simulink model "INTMRStateCtrl"  (R2018b)
settings: Solver=FixedStepDiscrete  StartTime=0.0  StopTime=10.0  FixedStep=0.01  RelTol=1e-3
libraries: StateCtrlLib x1
settings Model: Creator=sn2xws  LastModifiedBy=sn2xws
settings DataIOCC: SaveFormat=StructureWithTime
settings OptimizationCC: DefaultParameterBehavior=Inlined  EnhancedBackFolding=on  PassReuseOutputArgsAs=Individual arguments  ZeroExternalMemoryAtStartup=off  ZeroInternalMemoryAtStartup=off  OptimizeBlockOrder=speed  DifferentSizesBufferReuse=on  OptimizationCustomize=off
settings DebuggingCC: ParameterTunabilityLossMsg=error
settings ModelReferenceCC: ModelReferenceNumInstancesAllowed=Single
settings SFSimCC: MATLABDynamicMemAlloc=off
settings RTWCC: SystemTargetFile=autosar.tlc  GenCodeOnly=on  TemplateMakefile=ert_default_tmf  Description=AUTOSAR  GenerateReport=on  IncludeHyperlinkInReport=on  LaunchReport=on  GenerateTraceInfo=on  GenerateTraceReport=on  GenerateTraceReportSl=on  GenerateTraceReportSf=on  GenerateTraceReportEml=on
settings CodeAppCC: ForceParamTrailComments=on  IgnoreCustomStorageClasses=off  OperatorAnnotations=on  SimulinkDataObjDesc=on  SFDataObjDesc=on  InsertBlockDesc=on
settings STFCustomTargetCC: TargetLangStandard=C99 (ISO)  MultiwordLength=256  ParMdlRefBuildCompliant=on  CompOptLevelCompliant=on  IncludeMdlTerminateFcn=off  CombineOutputUpdateFcns=on  SuppressErrorStatus=on  ERTCustomFileBanners=on  SupportNonFinite=off  SupportComplex=off  SupportContinuousTime=off  SupportNonInlinedSFcns=off  RemoveResetFunc=on  MATLABClassNameForMDSCustomization=Simulink.SoftwareTarget.ERTCustomization  AutosarCompliant=on  UseToolchainInfoCompliant=on  LookupTableObjectStructAxisOrder=2,1,3,4,...  LUTObjectStructOrderEvenSpacing=Size,Table,Breakpoints  SystemTargetFile=autosar.tlc
settings ERTTargetCC: TargetLangStandard=C99 (ISO)  ConcurrentExecutionCompliant=off  IncludeMdlTerminateFcn=off  SuppressErrorStatus=on  SupportNonFinite=off  SupportComplex=off  ModelStepFunctionPrototypeControlCompliant=off  CPPClassGenCompliant=off  AutosarCompliant=on  LookupTableObjectStructAxisOrder=2,1,3,4,...  LUTObjectStructOrderEvenSpacing=Size,Table,Breakpoints  InlinedParameterPlacement=NonHierarchical  ERTCustomFileTemplate=example_file_process.tlc

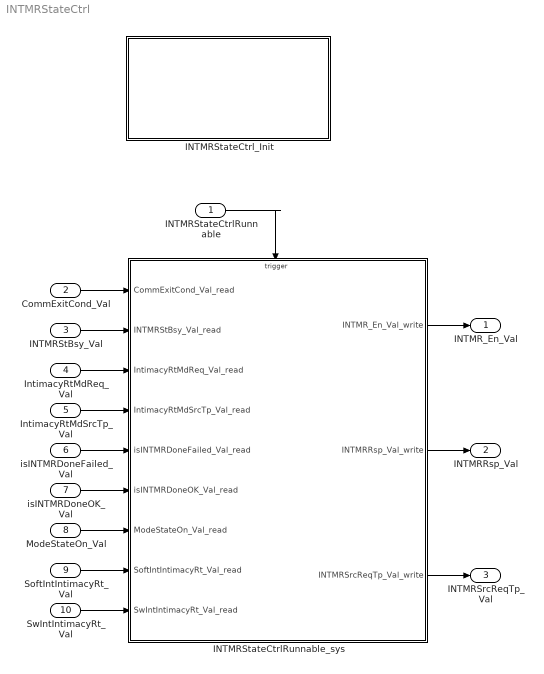
== system INTMRStateCtrl ==
  INTMRStateCtrlRunnable : Inport  SampleTime=0.01  OutputFunctionCall=on
  CommExitCond_Val : Inport  Port=2  OutDataTypeStr=boolean  PortDimensions=1
  INTMRStBsy_Val : Inport  Port=3  OutDataTypeStr=boolean  PortDimensions=1
  IntimacyRtMdReq_Val : Inport  Port=4  OutDataTypeStr=boolean  PortDimensions=1
  IntimacyRtMdSrcTp_Val : Inport  Port=5  OutDataTypeStr=Enum: SrcReqTp1  PortDimensions=1
  isINTMRDoneFailed_Val : Inport  Port=6  OutDataTypeStr=boolean  PortDimensions=1
  isINTMRDoneOK_Val : Inport  Port=7  OutDataTypeStr=boolean  PortDimensions=1
  ModeStateOn_Val : Inport  Port=8  OutDataTypeStr=boolean  PortDimensions=1
  SoftIntIntimacyRt_Val : Inport  Port=9  OutDataTypeStr=IntEnable  PortDimensions=1
  SwIntIntimacyRt_Val : Inport  Port=10  OutDataTypeStr=IntEnable  PortDimensions=1
  INTMRStateCtrlRunnable_sys : Subsystem
  INTMRStateCtrl_Init : Subsystem
  INTMR_En_Val : Outport  OutDataTypeStr=boolean  PortDimensions=1
  INTMRRsp_Val : Outport  Port=2  OutDataTypeStr=Enum: MdRspLocal1  PortDimensions=1
  INTMRSrcReqTp_Val : Outport  Port=3  OutDataTypeStr=Enum: SrcReqTp1  PortDimensions=1
  wires:
  CommExitCond_Val/1 -> INTMRStateCtrlRunnable_sys/1(CommExitCond_Val_read)
  INTMRStBsy_Val/1 -> INTMRStateCtrlRunnable_sys/2(INTMRStBsy_Val_read)
  IntimacyRtMdReq_Val/1 -> INTMRStateCtrlRunnable_sys/3(IntimacyRtMdReq_Val_read)
  IntimacyRtMdSrcTp_Val/1 -> INTMRStateCtrlRunnable_sys/4(IntimacyRtMdSrcTp_Val_read)
  isINTMRDoneFailed_Val/1 -> INTMRStateCtrlRunnable_sys/5(isINTMRDoneFailed_Val_read)
  isINTMRDoneOK_Val/1 -> INTMRStateCtrlRunnable_sys/6(isINTMRDoneOK_Val_read)
  ModeStateOn_Val/1 -> INTMRStateCtrlRunnable_sys/7(ModeStateOn_Val_read)
  SoftIntIntimacyRt_Val/1 -> INTMRStateCtrlRunnable_sys/8(SoftIntIntimacyRt_Val_read)
  SwIntIntimacyRt_Val/1 -> INTMRStateCtrlRunnable_sys/9(SwIntIntimacyRt_Val_read)
  INTMRStateCtrlRunnable_sys/1(INTMR_En_Val_write) -> INTMR_En_Val/1
  INTMRStateCtrlRunnable_sys/2(INTMRRsp_Val_write) -> INTMRRsp_Val/1
  INTMRStateCtrlRunnable_sys/3(INTMRSrcReqTp_Val_write) -> INTMRSrcReqTp_Val/1
  INTMRStateCtrlRunnable/1 -> INTMRStateCtrlRunnable_sys/Trigger

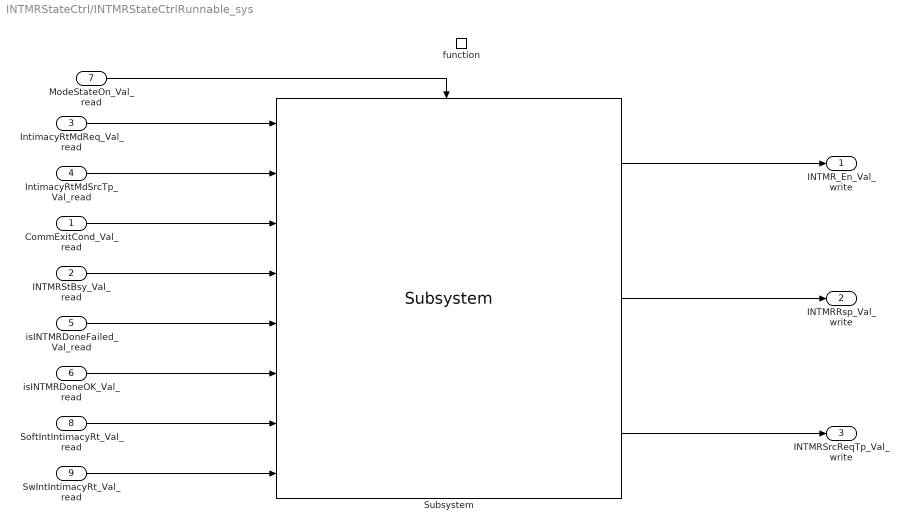
== system INTMRStateCtrl/INTMRStateCtrlRunnable_sys ==
  CommExitCond_Val_read : Inport
  INTMRStBsy_Val_read : Inport  Port=2
  IntimacyRtMdReq_Val_read : Inport  Port=3
  IntimacyRtMdSrcTp_Val_read : Inport  Port=4
  isINTMRDoneFailed_Val_read : Inport  Port=5
  isINTMRDoneOK_Val_read : Inport  Port=6
  ModeStateOn_Val_read : Inport  Port=7
  SoftIntIntimacyRt_Val_read : Inport  Port=8
  SwIntIntimacyRt_Val_read : Inport  Port=9
  function : TriggerPort  TriggerType=function-call  VariantControl=(inherit)  SampleTimeType=periodic  SampleTime=-1
  Subsystem : StateCtrlLib/Subsystem  SystemSampleTime=-1
  INTMR_En_Val_write : Outport
      settings: EnsureOutportIsVirtual=on
  INTMRRsp_Val_write : Outport  Port=2
      settings: EnsureOutportIsVirtual=on
  INTMRSrcReqTp_Val_write : Outport  Port=3
      settings: EnsureOutportIsVirtual=on
  wires:
  ModeStateOn_Val_read/1 -> Subsystem/Enable
  IntimacyRtMdReq_Val_read/1 -> Subsystem/1
  IntimacyRtMdSrcTp_Val_read/1 -> Subsystem/2
  CommExitCond_Val_read/1 -> Subsystem/3
  INTMRStBsy_Val_read/1 -> Subsystem/4
  SoftIntIntimacyRt_Val_read/1 -> Subsystem/7
  isINTMRDoneFailed_Val_read/1 -> Subsystem/5
  SwIntIntimacyRt_Val_read/1 -> Subsystem/8
  isINTMRDoneOK_Val_read/1 -> Subsystem/6
  Subsystem/1 -> INTMR_En_Val_write/1
  Subsystem/2 -> INTMRRsp_Val_write/1
  Subsystem/3 -> INTMRSrcReqTp_Val_write/1

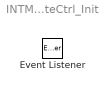
== system INTMRStateCtrl/INTMRStateCtrl_Init ==
  Event Listener : EventListener  EventName=reset
